simulink model "rtwdemo_ssreuse"  (Simulink 6.0)
settings: Solver=FixedStepDiscrete  StartTime=0.0  StopTime=10.0  RelTol=1e-3
PreLoadFcn:
  | rtwdemo_ssreuse_data
values from neighbouring files (symbols this model uses):
  T1Break = Simulink.Parameter    [rtwdemo_exprfolding_data.m]    (also in rtwdemo_paraminline_data.m; rtwdemo_ssreuse_data.m)
  T1Data = Simulink.Parameter    [rtwdemo_exprfolding_data.m]    (also in rtwdemo_paraminline_data.m; rtwdemo_ssreuse_data.m)
  T2Break = Simulink.Parameter    [rtwdemo_exprfolding_data.m]    (also in rtwdemo_paraminline_data.m; rtwdemo_ssreuse_data.m = copy(T1Break))
  T2Data = Simulink.Parameter    [rtwdemo_exprfolding_data.m]    (also in rtwdemo_paraminline_data.m; rtwdemo_ssreuse_data.m = copy(T1Data))
libraries: rtwdemowidgets x2
settings Model: Creator=The MathWorks Inc.  LastModifiedBy=batserve  ExtModeAutoUpdateStatusClock=off
settings DataIOCC: SaveOutput=off  SaveTime=off  SignalLoggingName=sigsOut
settings OptimizationCC: InlineParams=on  EnforceIntegerDowncast=off  StateBitsets=on  DataBitsets=on  UseTempVars=on
settings DebuggingCC: CheckExecutionContextPreStartOutputMsg=on  CheckExecutionContextRuntimeOutputMsg=on  SolverPrmCheckMsg=none
settings RTWCC: TLCOptions=-p0 -aWarnNonSaturatedBlocks=0  GenerateReport=on  RTWVerbose=off  ProcessScript=grt_make_rtw_hook  LaunchReport=on
settings CodeAppCC: ForceParamTrailComments=on  PrefixModelToSubsysFcnNames=off
settings GRTTargetCC: MatFileLogging=off

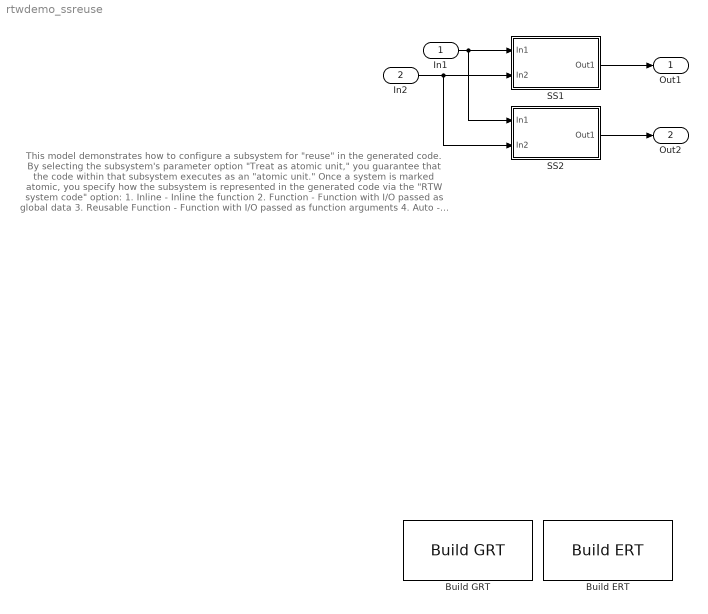
== system rtwdemo_ssreuse ==
  note: This model demonstrates how to configure a subsystem for "reuse" in the generated code.  By selecting the
      | subsystem's parameter option "Treat as atomic unit," you guarantee that the code within that subsystem
      | executes as an "atomic unit."  Once a system is marked atomic, you specify how the subsystem is represented
      | in the generated code via the "RTW system code" option:
      |
      | 1. Inline            - Inline the function
      | 2. Function          - Function with I/O passed as global data
      | 3. Reusable Function - Function with I/O passed as function arguments
      | 4. Auto              - Let RTW optimize based on context
      |
      | Cases 3 and 4 permit Simulink to reuse the subsystem in the generated code.  The function name is controlled
      | with the "RTW function name" option.  Here, SS2 is simply a copy of SS1, which is configured as a "Reusable
      | Function" with function name "myfun."  Notice that the system is a parameterized masked subsystem.  Parameters
      | of a mask become arguments to the function.  This example specifies T1Break, T2Data, T2Break, and T2Data
      | parameters.
      |
      | To see the subsystem parameters settings, right-click on the subsystem block and select "SubSystem
      | Parameters..."
      |
      | To see the content of the masked subsystem, right-click on the subsystem block and select "Look Under Mask."
  In1 : Inport  Port=1  LatchInput=off
  In2 : Inport  Port=2  LatchInput=off
  Build ERT : rtwdemowidgets/Build ERT  attrib_overrides={}
  Build GRT : rtwdemowidgets/Build GRT  attrib_overrides={}
  SS1 : Subsystem  TreatAsAtomicUnit=on  PropExecContextAcrossSSBoundary=on  RTWFcnName=myfun  RTWFileName=myfile  mask(SSDemo){x=T1Break, y=T1Data}
      mask prompts: x "Break points (X data):"; y "Output values (Y data):"
      mask help: Example to demonstrate code reuse. This example has two parameters for a lookup table.
      settings: RTWFcnNameOpts=User specified
  SS2 : Subsystem  TreatAsAtomicUnit=on  PropExecContextAcrossSSBoundary=on  RTWFcnName=myfun  RTWFileName=myfile  mask(SSDemo){x=T2Break, y=T2Data}
      mask prompts: x "Break points (X data):"; y "Output values (Y data):"
      mask help: Example to demonstrate code reuse. This example has two parameters for a lookup table.
      settings: RTWFcnNameOpts=User specified
  Out1 : Outport
  Out2 : Outport  Port=2
  wires:
  SS1/1(Out1) -> Out1/1
  In2/1 -> SS1/2(In2), SS2/2(In2)
  In1/1 -> SS1/1(In1), SS2/1(In1)
  SS2/1(Out1) -> Out2/1

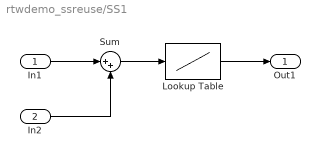
== system rtwdemo_ssreuse/SS1 ==
  In1 : Inport  Port=1  LatchInput=off
  In2 : Inport  Port=2  LatchInput=off
  Lookup Table : Lookup  DialogController=Simulink.DDGSource  InputValues=x  OutputValues=y
  Sum : Sum  Inputs=|++
  Out1 : Outport
  wires:
  In1/1 -> Sum/1
  Lookup Table/1 -> Out1/1
  In2/1 -> Sum/2
  Sum/1 -> Lookup Table/1

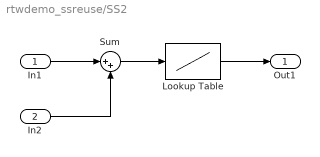
== system rtwdemo_ssreuse/SS2 ==
  In1 : Inport  Port=1  LatchInput=off
  In2 : Inport  Port=2  LatchInput=off
  Lookup Table : Lookup  DialogController=Simulink.DDGSource  InputValues=x  OutputValues=y
  Sum : Sum  Inputs=|++
  Out1 : Outport
  wires:
  Sum/1 -> Lookup Table/1
  In2/1 -> Sum/2
  Lookup Table/1 -> Out1/1
  In1/1 -> Sum/1
